simulink model "rgb2gray"  (Simulink 7.4)
settings: Solver=VariableStepDiscrete  StartTime=0.0  StopTime=20  RelTol=1e-3
libraries: xbsIndex_r4 x15, xbsCopyrightNotice_r4 x1
settings Model: Creator=jou  LastModifiedBy=douangp
settings DataIOCC: SignalLoggingName=sigsOut
settings OptimizationCC: InlineInvariantSignals=on  InitFltsAndDblsToZero=on
settings DebuggingCC: SaveWithParameterizedLinksMsg=none  SignalResolutionControl=TryResolveAllWithWarning  SolverPrmCheckMsg=none  MultiTaskDSMMsg=warning  MultiTaskCondExecSysMsg=none  StrictBusMsg=None
settings HardwareCC: TargetUnknown=on
settings RTWCC: IncludeERTFirstTime=on
settings GRTTargetCC: TargetFcnLib=ansi_tfl_tmw.mat

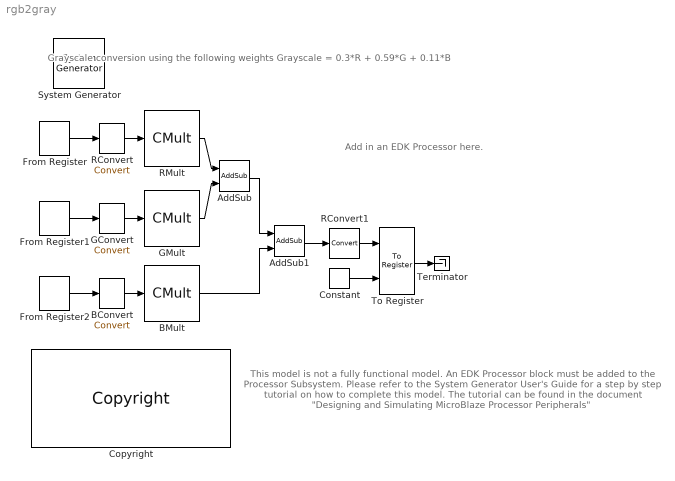
== system rgb2gray ==
  note: Grayscale conversion using the following weights
      | Grayscale = 0.3*R + 0.59*G + 0.11*B
  note: Add in an EDK Processor here.
  note: This model is not a fully functional model. An EDK Processor block must
      | be added to the  Processor Subsystem.
      |
      | Please refer to the System Generator User's Guide for a step by step
      | tutorial on how to complete this model. The tutorial can be found
      | in the document "Designing and Simulating MicroBlaze Processor Peripherals"
  " System Generator" : xbsIndex_r4/ System Generator  Tag=genX  SystemSampleTime=-1  xilinxfamily=virtex6  part=xc6vsx315t  speed=-3  package=ff1156  synthesis_tool=XST  clock_wrapper=Clock Enables  directory=./netlist  testbench=off  simulink_period=1  sysclk_period=10  dcm_input_clock_period=10  incr_netlist=off  trim_vbits=Everywhere in SubSystem  dbl_ovrd=According to Block Masks  core_generation=According to Block Masks  run_coregen=off  deprecated_control=off  eval_field=0  block_type=sysgen
      settings: block_version=12.2
  AddSub : xbsIndex_r4/AddSub  mode=Addition  use_carryin=off  use_carryout=off  en=off  latency=1  precision=Full  arith_type=Unsigned  n_bits=8  bin_pt=2  quantization=Truncate  overflow=Wrap  dbl_ovrd=off  use_behavioral_HDL=on  hw_selection=Fabric  pipelined=off  use_rpm=on  block_type=addsub
      settings: xl_area=[0, 0, 0, 0, 0, 0, 0]  block_version=VER_STRING_GOES_HERE
  AddSub1 : xbsIndex_r4/AddSub  mode=Addition  use_carryin=off  use_carryout=off  en=off  latency=0  precision=Full  arith_type=Unsigned  n_bits=8  bin_pt=2  quantization=Truncate  overflow=Wrap  dbl_ovrd=off  use_behavioral_HDL=on  hw_selection=Fabric  pipelined=off  use_rpm=on  block_type=addsub
      settings: xl_area=[0, 0, 0, 0, 0, 0, 0]  block_version=VER_STRING_GOES_HERE
  BConvert : xbsIndex_r4/Convert  arith_type=Unsigned  n_bits=16  bin_pt=8  quantization=Truncate  overflow=Wrap  en=off  latency=0  dbl_ovrd=off  pipeline=off  block_type=convert
      settings: xl_area=[0, 0, 0, 0, 0, 0, 0]  block_version=VER_STRING_GOES_HERE
  BMult : xbsIndex_r4/CMult  const=0.11  const_n_bits=16  const_bin_pt=8  en=off  latency=0  precision=Full  arith_type="Signed  (2's comp)"  n_bits=8  bin_pt=6  quantization="Round  (unbiased: +/- Inf)"  overflow=Wrap  dbl_ovrd=off  use_behavioral_HDL=off  mem_type=Distributed RAM  pipeline=off  use_rpm=on  placement_style=Rectangular Shape  block_type=cmult
      settings: xl_area=[0, 0, 0, 0, 0, 0, 0]  block_version=VER_STRING_GOES_HERE
  Constant : xbsIndex_r4/Constant  arith_type=Boolean  const=1  n_bits=16  bin_pt=14  explicit_period=on  period=1  equ=P=C  opselect=C  inp2=PCIN>>17  opr=+  inp1=P  carry=CIN  dbl_ovrd=off  block_type=constant
      settings: block_version=VER_STRING_GOES_HERE
  Copyright : xbsCopyrightNotice_r4/Copyright  copyrighttext="Copyright (c) 2010  by  Xilinx, Inc. All rights reserved.<br><br>This file contains proprietary, confidential information of Xilinx, Inc., is distributed under licensefrom Xilinx, Inc., and may be used, copied and/or disclosed only pursuant to the terms of a valid licenseagreement with Xilinx, Inc. Xilinx hereby grants you a license to use this file solely for design,simulation, implementation and creation of design files limited to Xilinx devices or technologies. Use with non-Xilinx devices or technologies is expressly prohibited and immediately terminates your license unless covered by a separate agreement.<br><br>Xilinx is providing this design, code, or information \"as-is\" solely for use in developing programs and solutions for Xilinx devices, with no obligation on the part of Xilinx to provide support. By providingthis design, code, or information as one possible implementation of this feature, application or standard,Xilinx is making no representation that this implementation is free from any claims of infringement. Youare responsible for obtaining any rights you may require for your implementation. Xilinx expressly disclaimsany warranty whatsoever with respect to the adequacy of the implementation, including but not limited to anywarranties or representations that this implementation is free from claims of infringement, implied warrantiesof merchantability or fitness for a particular purpose.<br><br>Xilinx products are not intended for use in life support appliances, devices, or systems. Use in such applications is expressly prohibited.<br><br>Any modifications that are made to the Source Code are done at the user's sole risk and will be unsupported.<br><br>This copyright and support notice must be retained as part of this text at all times. (c) Copyright 1995-2010 Xilinx, Inc. All rights reserved."  block_type=copyright
      settings: block_version=10.1.00
      settings: infoedit=|
      | Copyright(C) 2007 by  Xilinx, Inc. All rights reserved.<br>
      | <br>
      | This file contains proprietary, confidential information of Xilinx, Inc., is distributed under license
      | from Xilinx, Inc., and may be used, copied and/or disclosed only pursuant to the terms of a valid license
      | agreement with Xilinx, Inc. Xilinx hereby grants you a license to use this file solely for design,
      | simulation, implementation and creation of design files limited to Xilinx devices or technologies. Use
      | with non-Xilinx devices or technologies is expressly prohibited and immediately terminates your license
      | unless covered by a separate agreement.<br>
      | <br>
      | Xilinx is providing this design, code, or information "as-is" solely for use in developing programs and
      | solutions for Xilinx devices, with no obligation on the part of Xilinx to provide support. By providing
      | this design, code, or information as one possible implementation of this feature, application or standard,
      | Xilinx is making no representation that this implementation is free from any claims of infringement. You
      | are responsible for obtaining any rights you may require for your implementation. Xilinx expressly disclaims
      | any warranty whatsoever with respect to the adequacy of the implementation, including but not limited to any
      | warranties or representations that this implementation is free from claims of infringement, implied warranties
      | of merchantability or fitness for a particular purpose.<br>
      | <br>
      | Xilinx products are not intended for use in life support appliances, devices, or systems. Use in such
      | applications is expressly prohibited.<br>
      | <br>
      | Any modifications that are made to the Source Code are done at the user's sole risk and will be unsupported.<br>
      | <br>
      | This copyright and support notice must be retained as part of this text at all times.
      | (c) Copyright 1995-2007 Xilinx, Inc. All rights reserved.
  From Register : xbsIndex_r4/From Register  shared_memory_name='red'  init=0  period=1  ownership=Owned and initialized elsewhere  arith_type=Unsigned  n_bits=8  bin_pt=0  dbl_ovrd=off  block_type=fromreg
      settings: AttributesFormatString=<< %<shared_memory_name> >>  infoedit="Register block that reads data to a shared memory register.  Delay of one sample period."  block_version=VER_STRING_GOES_HERE
  From Register1 : xbsIndex_r4/From Register  shared_memory_name='green'  init=0  period=1  ownership=Owned and initialized elsewhere  arith_type=Unsigned  n_bits=8  bin_pt=0  dbl_ovrd=off  block_type=fromreg
      settings: AttributesFormatString=<< %<shared_memory_name> >>  infoedit="Register block that reads data to a shared memory register.  Delay of one sample period."  block_version=VER_STRING_GOES_HERE
  From Register2 : xbsIndex_r4/From Register  shared_memory_name='blue'  init=0  period=1  ownership=Owned and initialized elsewhere  arith_type=Unsigned  n_bits=8  bin_pt=0  dbl_ovrd=off  block_type=fromreg
      settings: AttributesFormatString=<< %<shared_memory_name> >>  infoedit="Register block that reads data to a shared memory register.  Delay of one sample period."  block_version=VER_STRING_GOES_HERE
  GConvert : xbsIndex_r4/Convert  arith_type=Unsigned  n_bits=16  bin_pt=8  quantization=Truncate  overflow=Wrap  en=off  latency=0  dbl_ovrd=off  pipeline=off  block_type=convert
      settings: xl_area=[0, 0, 0, 0, 0, 0, 0]  block_version=VER_STRING_GOES_HERE
  GMult : xbsIndex_r4/CMult  const=0.59  const_n_bits=16  const_bin_pt=8  en=off  latency=0  precision=Full  arith_type="Signed  (2's comp)"  n_bits=8  bin_pt=6  quantization="Round  (unbiased: +/- Inf)"  overflow=Wrap  dbl_ovrd=off  use_behavioral_HDL=off  mem_type=Distributed RAM  pipeline=off  use_rpm=on  placement_style=Rectangular Shape  block_type=cmult
      settings: xl_area=[0, 0, 0, 0, 0, 0, 0]  block_version=VER_STRING_GOES_HERE
  RConvert : xbsIndex_r4/Convert  arith_type=Unsigned  n_bits=16  bin_pt=8  quantization=Truncate  overflow=Wrap  en=off  latency=0  dbl_ovrd=off  pipeline=off  block_type=convert
      settings: xl_area=[0, 0, 0, 0, 0, 0, 0]  block_version=VER_STRING_GOES_HERE
  RConvert1 : xbsIndex_r4/Convert  arith_type=Unsigned  n_bits=32  bin_pt=0  quantization=Truncate  overflow=Wrap  en=off  latency=0  dbl_ovrd=off  pipeline=off  block_type=convert
      settings: xl_area=[0, 0, 0, 0, 0, 0, 0]  block_version=VER_STRING_GOES_HERE
  RMult : xbsIndex_r4/CMult  const=0.3  const_n_bits=16  const_bin_pt=8  en=off  latency=0  precision=Full  arith_type="Signed  (2's comp)"  n_bits=8  bin_pt=6  quantization="Round  (unbiased: +/- Inf)"  overflow=Wrap  dbl_ovrd=off  use_behavioral_HDL=off  mem_type=Distributed RAM  pipeline=off  use_rpm=on  placement_style=Rectangular Shape  block_type=cmult
      settings: xl_area=[0, 0, 0, 0, 0, 0, 0]  block_version=VER_STRING_GOES_HERE
  Terminator : Terminator
  To Register : xbsIndex_r4/To Register  shared_memory_name='result'  init=0  ownership=Locally owned and initialized  explicit_data_type=on  arith_type=Unsigned  n_bits=32  bin_pt=0  dbl_ovrd=off  block_type=toreg
      settings: AttributesFormatString=<< %<shared_memory_name> >>  infoedit="Register block that writes data to a shared memory register.  Delay of one sample period."  block_version=VER_STRING_GOES_HERE
  wires:
  AddSub/1 -> AddSub1/1
  GMult/1 -> AddSub/2
  RMult/1 -> AddSub/1
  BConvert/1 -> BMult/1
  From Register2/1 -> BConvert/1
  GConvert/1 -> GMult/1
  From Register1/1 -> GConvert/1
  From Register/1 -> RConvert/1
  RConvert/1 -> RMult/1
  BMult/1 -> AddSub1/2
  AddSub1/1 -> RConvert1/1
  RConvert1/1 -> To Register/1
  Constant/1 -> To Register/2
  To Register/1 -> Terminator/1
